simulink model "gm_lab1"  (R2022a)
settings: Solver=FixedStepAuto  StartTime=0.0  StopTime=1e6  RelTol=1e-3
settings Model: Creator=user  LastModifiedBy=user
settings OptimizationCC: BlockReduction=off  ConditionallyExecuteInputs=off
settings DebuggingCC: InheritedTsInSrcMsg=none

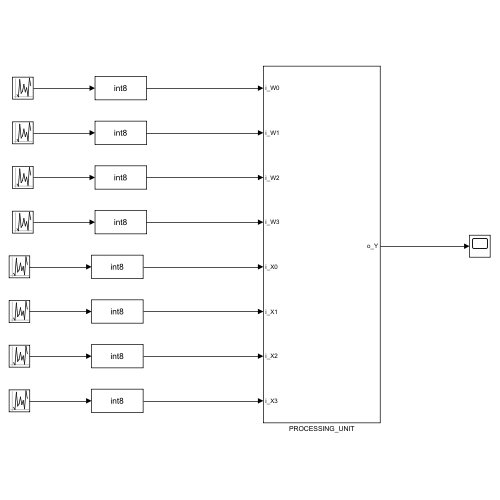
[thumbnail: Simulink's stored preview of the top-level diagram]
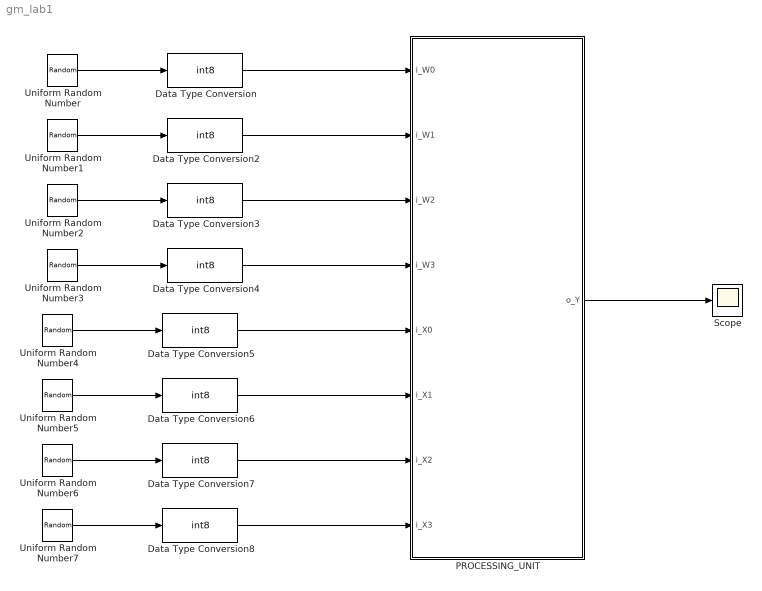
== system gm_lab1 ==
  Data Type Conversion{,2..8} (8 alike) : DataTypeConversion  OutDataTypeStr=int8  SaturateOnIntegerOverflow=off  RndMeth=Floor
  PROCESSING_UNIT : Subsystem
  Scope : Scope
  Uniform Random Number : UniformRandomNumber  Minimum=-2^7  Maximum=2^7-1  Seed=11  SampleTime=1
  Uniform Random Number1 : UniformRandomNumber  Minimum=-2^7  Maximum=2^7-1  Seed=12  SampleTime=1
  Uniform Random Number2 : UniformRandomNumber  Minimum=-2^7  Maximum=2^7-1  Seed=13  SampleTime=1
  Uniform Random Number3 : UniformRandomNumber  Minimum=-2^7  Maximum=2^7-1  Seed=14  SampleTime=1
  Uniform Random Number4 : UniformRandomNumber  Minimum=-2^7  Maximum=2^7-1  Seed=15  SampleTime=1
  Uniform Random Number5 : UniformRandomNumber  Minimum=-2^7  Maximum=2^7-1  Seed=16  SampleTime=1
  Uniform Random Number6 : UniformRandomNumber  Minimum=-2^7  Maximum=2^7-1  Seed=17  SampleTime=1
  Uniform Random Number7 : UniformRandomNumber  Minimum=-2^7  Maximum=2^7-1  Seed=18  SampleTime=1
  wires:
  PROCESSING_UNIT/1(o_Y) -> Scope/1
  Data Type Conversion8/1 -> PROCESSING_UNIT/8(i_X3)
  Data Type Conversion7/1 -> PROCESSING_UNIT/7(i_X2)
  Data Type Conversion6/1 -> PROCESSING_UNIT/6(i_X1)
  Data Type Conversion5/1 -> PROCESSING_UNIT/5(i_X0)
  Data Type Conversion/1 -> PROCESSING_UNIT/1(i_W0)
  Data Type Conversion2/1 -> PROCESSING_UNIT/2(i_W1)
  Data Type Conversion3/1 -> PROCESSING_UNIT/3(i_W2)
  Data Type Conversion4/1 -> PROCESSING_UNIT/4(i_W3)
  Uniform Random Number7/1 -> Data Type Conversion8/1
  Uniform Random Number6/1 -> Data Type Conversion7/1
  Uniform Random Number5/1 -> Data Type Conversion6/1
  Uniform Random Number4/1 -> Data Type Conversion5/1
  Uniform Random Number3/1 -> Data Type Conversion4/1
  Uniform Random Number2/1 -> Data Type Conversion3/1
  Uniform Random Number1/1 -> Data Type Conversion2/1
  Uniform Random Number/1 -> Data Type Conversion/1

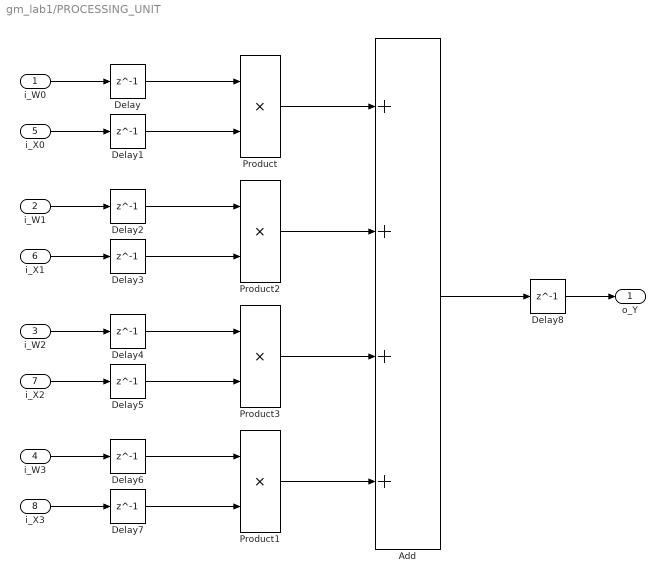
== system gm_lab1/PROCESSING_UNIT ==
  i_W0 : Inport
  i_W1 : Inport  Port=2
  i_W2 : Inport  Port=3
  i_W3 : Inport  Port=4
  i_X0 : Inport  Port=5
  i_X1 : Inport  Port=6
  i_X2 : Inport  Port=7
  i_X3 : Inport  Port=8
  Add : Sum  Inputs=++++
  Delay{,1..8} (9 alike) : Delay  DelayLength=1  InitialCondition=0  SampleTime=1
  Product{,1..3} (4 alike) : Product
  o_Y : Outport
  wires:
  Delay8/1 -> o_Y/1
  Delay7/1 -> Product1/2
  Delay6/1 -> Product1/1
  Delay5/1 -> Product3/2
  Delay4/1 -> Product3/1
  Delay3/1 -> Product2/2
  Delay2/1 -> Product2/1
  Delay1/1 -> Product/2
  Delay/1 -> Product/1
  Product1/1 -> Add/4
  i_X3/1 -> Delay7/1
  i_W3/1 -> Delay6/1
  i_X2/1 -> Delay5/1
  i_W2/1 -> Delay4/1
  Product3/1 -> Add/3
  Product2/1 -> Add/2
  i_X0/1 -> Delay1/1
  i_X1/1 -> Delay3/1
  i_W1/1 -> Delay2/1
  i_W0/1 -> Delay/1
  Product/1 -> Add/1
  Add/1 -> Delay8/1
